simulink model "assignments_week6"  (R2024b)
settings: Solver=VariableStepAuto  StartTime=0.0  StopTime=20  RelTol=1e-3
model workspace (MAT data in the model file):
  C = 1
  L = 1
  R = 0.25
settings Model: Creator=marti  LastModifiedBy=marti

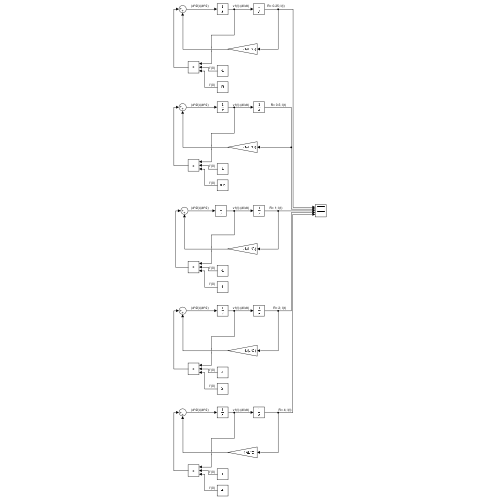
[thumbnail: Simulink's stored preview of the top-level diagram]
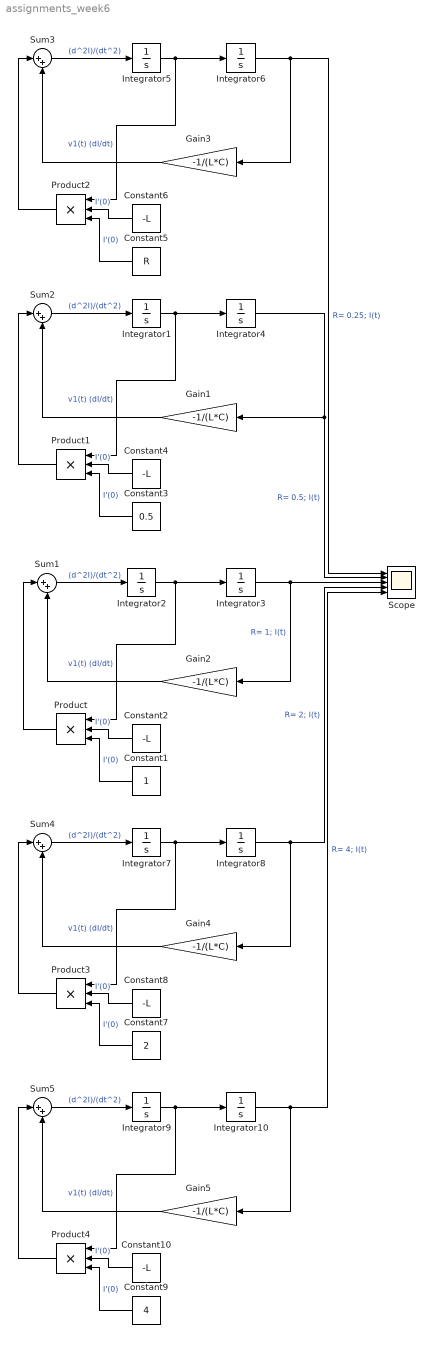
== system assignments_week6 ==
  Constant1 : Constant
  Constant{2,4,6,8,10} (5 alike) : Constant  Value=-L
  Constant3 : Constant  Value=0.5
  Constant5 : Constant  Value=R
  Constant7 : Constant  Value=2
  Constant9 : Constant  Value=4
  Gain{1..5} (5 alike) : Gain  Gain=-1/(L*C)
  Integrator{1..2,5,7,9} (5 alike) : Integrator  InitialCondition=4
  Integrator{3..4,6,8,10} (5 alike) : Integrator
  Product{,1..4} (5 alike) : Product  Inputs=3
  Scope : Scope  NumInputPorts=5
  Sum{1..5} (5 alike) : Sum  Inputs=|++
  wires:
  Integrator2/1 -> Product/1, Integrator3/1  "v1(t) (dI/dt)"
  Sum1/1 -> Integrator2/1  "(d^2I)/(dt^2)"
  Integrator3/1 -> Gain2/1, Scope/3  "R= 1; I(t)"
  Gain2/1 -> Sum1/2
  Constant2/1 -> Product/2  "I'(0)"
  Product/1 -> Sum1/1
  Constant1/1 -> Product/3  "I'(0)"
  Constant3/1 -> Product1/3  "I'(0)"
  Integrator1/1 -> Product1/1, Integrator4/1  "v1(t) (dI/dt)"
  Integrator4/1 -> Gain1/1, Scope/2  "R= 0.5; I(t)"
  Sum2/1 -> Integrator1/1  "(d^2I)/(dt^2)"
  Product1/1 -> Sum2/1
  Constant4/1 -> Product1/2  "I'(0)"
  Gain1/1 -> Sum2/2
  Constant5/1 -> Product2/3  "I'(0)"
  Integrator5/1 -> Product2/1, Integrator6/1  "v1(t) (dI/dt)"
  Integrator6/1 -> Scope/1, Gain3/1  "R= 0.25; I(t)"
  Sum3/1 -> Integrator5/1  "(d^2I)/(dt^2)"
  Product2/1 -> Sum3/1
  Constant6/1 -> Product2/2  "I'(0)"
  Gain3/1 -> Sum3/2
  Constant7/1 -> Product3/3  "I'(0)"
  Integrator7/1 -> Product3/1, Integrator8/1  "v1(t) (dI/dt)"
  Integrator8/1 -> Scope/4, Gain4/1  "R= 2; I(t)"
  Sum4/1 -> Integrator7/1  "(d^2I)/(dt^2)"
  Product3/1 -> Sum4/1
  Constant8/1 -> Product3/2  "I'(0)"
  Gain4/1 -> Sum4/2
  Product4/1 -> Sum5/1
  Gain5/1 -> Sum5/2
  Constant10/1 -> Product4/2  "I'(0)"
  Constant9/1 -> Product4/3  "I'(0)"
  Integrator10/1 -> Scope/5, Gain5/1  "R= 4; I(t)"
  Integrator9/1 -> Product4/1, Integrator10/1  "v1(t) (dI/dt)"
  Sum5/1 -> Integrator9/1  "(d^2I)/(dt^2)"
